simulink model "mrefrobotarm_modified_previous_y_previous_ref"  (R2018b)
settings: Solver=FixedStepAuto  StartTime=0.0  StopTime=60  RelTol=1e-3  AbsTol=1e-6
undefined symbols (not defined in the file or in its folder): sfunxy2
libraries: neural x301, simulink x1
(part 9 of 10)

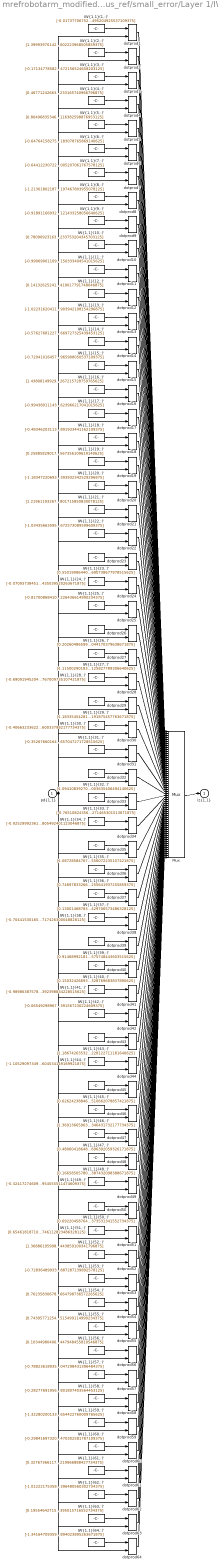
== system mrefrobotarm_modified_previous_y_previous_ref/small_error/Layer 1/IW{1,1} ==
  "pd{1,1}" : Inport  PortDimensions=8
      mask Display: e = 0.06;c1 = [120 230 180]/255;c2 = ([120 230 180]+0)/(256+128);c3 = ([120 230 180]+128)/(256+128);patch([0 1 1 0],[0 0 1 1],c1);patch([0 1 1 1-e 1-e 0+e],[0 0 1 1-e 0+e 0+e],c2);patch([0 0 1 1-e 0+e 0+e],[0 1 1 1-e 1-e 0+e],c3);plot([0 1 1 0 0],[0 0 1 1 0]);
  "IW{1,1}(1,:)'" : Constant  Value=[-0.017377067526509477890517274545345571823418140411376953125;-0.034011354582700097093361790712151560001075267791748046875;0.05439770936445220694821500728721730411052703857421875;-0.0629009283471842761681358524583629332482814788818359375;-2.987224863746458680680007091723382472991943359375;-0.2272943137249578138270322824610047973692417144775390625;0.038579930489393156334276824281914741732180118560791015625;-0.1025768959590427353845143443322740495204925537109375]
      mask Display: e = 0.06;c1 = [120 150 230]/255;c2 = ([120 150 230]+0)/383;c3 = ([120 150 230]+128)/383;patch([0 1 1 0],[0 0 1 1],c1);patch([0 1 1 1-e 1-e 0+e],[0 0 1 1-e 0+e 0+e],c2);patch([0 0 1 1-e 0+e 0+e],[0 1 1 1-e 1-e 0+e],c3);plot([0 1 1 0 0],[0 0 1 1 0]);disp('Weights');
  "IW{1,1}(10,:)'" : Constant  Value=[0.7809092316347172602064574675750918686389923095703125;0.09000232433482556471115998419918469153344631195068359375;-1.0678670373399123949553768397890962660312652587890625;-0.46394015522004983242965181489125825464725494384765625;-0.9896990789374815467027701743063516914844512939453125;-1.3552014415576343342451082207844592630863189697265625;-0.179686656791558874157743730393121950328350067138671875;-0.448255149939543795500895839722943492233753204345703125]
      mask Display: e = 0.06;c1 = [120 150 230]/255;c2 = ([120 150 230]+0)/383;c3 = ([120 150 230]+128)/383;patch([0 1 1 0],[0 0 1 1],c1);patch([0 1 1 1-e 1-e 0+e],[0 0 1 1-e 0+e 0+e],c2);patch([0 0 1 1-e 0+e 0+e],[0 1 1 1-e 1-e 0+e],c3);plot([0 1 1 0 0],[0 0 1 1 0]);disp('Weights');
  "IW{1,1}(11,:)'" : Constant  Value=[-0.99069001109756549272589154497836716473102569580078125;-0.10428566072279556176116699361955397762358188629150390625;0.55618964752205457546807565449853427708148956298828125;0.68297232673513941225706957993679679930210113525390625;-0.248998068763353452848008373621269129216670989990234375;0.644201394846871888688610852113924920558929443359375;1.25138751592991059879977910895831882953643798828125;-1.4140254443841655529467971064150333404541015625]
      mask Display: e = 0.06;c1 = [120 150 230]/255;c2 = ([120 150 230]+0)/383;c3 = ([120 150 230]+128)/383;patch([0 1 1 0],[0 0 1 1],c1);patch([0 1 1 1-e 1-e 0+e],[0 0 1 1-e 0+e 0+e],c2);patch([0 0 1 1-e 0+e 0+e],[0 1 1 1-e 1-e 0+e],c3);plot([0 1 1 0 0],[0 0 1 1 0]);disp('Weights');
  "IW{1,1}(12,:)'" : Constant  Value=[0.1413262524196326752612407062770216725766658782958984375;-0.6047035889340335312880370111088268458843231201171875;0.381641363428228796994545746201765723526477813720703125;0.84755222293533816202426578456652350723743438720703125;0.041896191821087412632262925171744427643716335296630859375;-1.3393596111062613385200847915257327258586883544921875;-1.16826698005478224473563386709429323673248291015625;-0.51017323607084985592763359818491153419017791748046875]
      mask Display: e = 0.06;c1 = [120 150 230]/255;c2 = ([120 150 230]+0)/383;c3 = ([120 150 230]+128)/383;patch([0 1 1 0],[0 0 1 1],c1);patch([0 1 1 1-e 1-e 0+e],[0 0 1 1-e 0+e 0+e],c2);patch([0 0 1 1-e 0+e 0+e],[0 1 1 1-e 1-e 0+e],c3);plot([0 1 1 0 0],[0 0 1 1 0]);disp('Weights');
  "IW{1,1}(13,:)'" : Constant  Value=[-1.0223162041134503663641908133286051452159881591796875;0.360795024277329456907636995310895144939422607421875;0.83528351858334992652288519821013323962688446044921875;-0.419973501162595186375625644359388388693332672119140625;-0.91936716478895308402030650540837086737155914306640625;-0.745110801710211045900678072939626872539520263671875;0.66761104678762228648025711663649417459964752197265625;1.0867368236477321641331172941136173903942108154296875]
      mask Display: e = 0.06;c1 = [120 150 230]/255;c2 = ([120 150 230]+0)/383;c3 = ([120 150 230]+128)/383;patch([0 1 1 0],[0 0 1 1],c1);patch([0 1 1 1-e 1-e 0+e],[0 0 1 1-e 0+e 0+e],c2);patch([0 0 1 1-e 0+e 0+e],[0 1 1 1-e 1-e 0+e],c3);plot([0 1 1 0 0],[0 0 1 1 0]);disp('Weights');
  "IW{1,1}(14,:)'" : Constant  Value=[-0.57627681227857741053099971395567990839481353759765625;0.857909167421744722759058277006261050701141357421875;-0.94860344887297232130407564909546636044979095458984375;-0.951059353750250746628580600372515618801116943359375;-0.08236091843453390015650228406229871325194835662841796875;-1.197742094847008775815311309997923672199249267578125;1.2108252364446354665261651462060399353504180908203125;0.157912941676574991589632190880365669727325439453125]
      mask Display: e = 0.06;c1 = [120 150 230]/255;c2 = ([120 150 230]+0)/383;c3 = ([120 150 230]+128)/383;patch([0 1 1 0],[0 0 1 1],c1);patch([0 1 1 1-e 1-e 0+e],[0 0 1 1-e 0+e 0+e],c2);patch([0 0 1 1-e 0+e 0+e],[0 1 1 1-e 1-e 0+e],c3);plot([0 1 1 0 0],[0 0 1 1 0]);disp('Weights');
  "IW{1,1}(15,:)'" : Constant  Value=[-0.7204101645789158236965477044577710330486297607421875;0.6308160303046788097702801678678952157497406005859375;0.423721818187184962045677139030885882675647735595703125;1.0038491536260936154434375566779635846614837646484375;-0.883054705141663287548681182670406997203826904296875;0.58133530731886706721667223973781801760196685791015625;-1.0898604085723462286949825283954851329326629638671875;0.75502926087022037560103626674390397965908050537109375]
      mask Display: e = 0.06;c1 = [120 150 230]/255;c2 = ([120 150 230]+0)/383;c3 = ([120 150 230]+128)/383;patch([0 1 1 0],[0 0 1 1],c1);patch([0 1 1 1-e 1-e 0+e],[0 0 1 1-e 0+e 0+e],c2);patch([0 0 1 1-e 0+e 0+e],[0 1 1 1-e 1-e 0+e],c3);plot([0 1 1 0 0],[0 0 1 1 0]);disp('Weights');
  "IW{1,1}(16,:)'" : Constant  Value=[1.4380814992902493099080629690433852374553680419921875;-0.76504143837121485471897130992147140204906463623046875;0.091006162532383749752540325062000192701816558837890625;1.083412609067099463544536774861626327037811279296875;-0.63205437136288289412533458744292147457599639892578125;-0.023231907766419000738178368692388175986707210540771484375;-0.38486268286379610170655496403924189507961273193359375;0.97191291146138658607611660045222379267215728759765625]
      mask Display: e = 0.06;c1 = [120 150 230]/255;c2 = ([120 150 230]+0)/383;c3 = ([120 150 230]+128)/383;patch([0 1 1 0],[0 0 1 1],c1);patch([0 1 1 1-e 1-e 0+e],[0 0 1 1-e 0+e 0+e],c2);patch([0 0 1 1-e 0+e 0+e],[0 1 1 1-e 1-e 0+e],c3);plot([0 1 1 0 0],[0 0 1 1 0]);disp('Weights');
  "IW{1,1}(17,:)'" : Constant  Value=[-0.99438911143919117563427789718843996524810791015625;1.1800184823356942853678219762514345347881317138671875;0.96225693879916296413767895501223392784595489501953125;0.92922137731835563467797101111500523984432220458984375;-0.165351050339907879038747751110349781811237335205078125;-0.92189358845869495695524165057577192783355712890625;-0.7329222503569459146177678121603094041347503662109375;-0.386713897740563139482361521004349924623966217041015625]
      mask Display: e = 0.06;c1 = [120 150 230]/255;c2 = ([120 150 230]+0)/383;c3 = ([120 150 230]+128)/383;patch([0 1 1 0],[0 0 1 1],c1);patch([0 1 1 1-e 1-e 0+e],[0 0 1 1-e 0+e 0+e],c2);patch([0 0 1 1-e 0+e 0+e],[0 1 1 1-e 1-e 0+e],c3);plot([0 1 1 0 0],[0 0 1 1 0]);disp('Weights');
  "IW{1,1}(18,:)'" : Constant  Value=[-0.48346203113266172923800922944792546331882476806640625;0.71561240921933866321325012904708273708820343017578125;0.2763669805789514821725560977938584983348846435546875;0.1785391777356719333891277301518130116164684295654296875;-1.282476848547498438080083360546268522739410400390625;-0.345188333939475733291857295625959523022174835205078125;-0.485833446458430129322181301176897250115871429443359375;0.37699947906613962000932360751903615891933441162109375]
      mask Display: e = 0.06;c1 = [120 150 230]/255;c2 = ([120 150 230]+0)/383;c3 = ([120 150 230]+128)/383;patch([0 1 1 0],[0 0 1 1],c1);patch([0 1 1 1-e 1-e 0+e],[0 0 1 1-e 0+e 0+e],c2);patch([0 0 1 1-e 0+e 0+e],[0 1 1 1-e 1-e 0+e],c3);plot([0 1 1 0 0],[0 0 1 1 0]);disp('Weights');
  "IW{1,1}(19,:)'" : Constant  Value=[0.25885829017035144605785035309963859617710113525390625;-0.75860387169028531406667070768889971077442169189453125;1.168586248003583794030646458850242197513580322265625;0.108415735019206482814269065784174017608165740966796875;-1.0403518157121827147904014054802246391773223876953125;0.227217134884770410874210710971965454518795013427734375;-0.1707771036802909758733903800020925700664520263671875;-1.05888387189785504460814991034567356109619140625]
      mask Display: e = 0.06;c1 = [120 150 230]/255;c2 = ([120 150 230]+0)/383;c3 = ([120 150 230]+128)/383;patch([0 1 1 0],[0 0 1 1],c1);patch([0 1 1 1-e 1-e 0+e],[0 0 1 1-e 0+e 0+e],c2);patch([0 0 1 1-e 0+e 0+e],[0 1 1 1-e 1-e 0+e],c3);plot([0 1 1 0 0],[0 0 1 1 0]);disp('Weights');
  "IW{1,1}(2,:)'" : Constant  Value=[1.399939701424660842832281559822149574756622314453125;1.1970420723626855608046071210992522537708282470703125;-1.2136352199150628461410406089271418750286102294921875;-0.52562314227074813377527107149944640696048736572265625;-0.04503930323055231610407389553074608556926250457763671875;0.83699176817769738168095727814943529665470123291015625;0.2363093463990357523396568240059423260390758514404296875;-0.244408544667858718124620054368278943002223968505859375]
      mask Display: e = 0.06;c1 = [120 150 230]/255;c2 = ([120 150 230]+0)/383;c3 = ([120 150 230]+128)/383;patch([0 1 1 0],[0 0 1 1],c1);patch([0 1 1 1-e 1-e 0+e],[0 0 1 1-e 0+e 0+e],c2);patch([0 0 1 1-e 0+e 0+e],[0 1 1 1-e 1-e 0+e],c3);plot([0 1 1 0 0],[0 0 1 1 0]);disp('Weights');
  "IW{1,1}(20,:)'" : Constant  Value=[-1.18347220693401045110704217222519218921661376953125;0.766009156958994186226163947139866650104522705078125;-1.0467062449262838352836979538551531732082366943359375;0.6851787478277435727846977897570468485355377197265625;-0.58848967369292604079333841582410968840122222900390625;0.8268949957131475070326587228919379413127899169921875;-0.8104681829608697540834327810443937778472900390625;0.20686385705200993623265048881876282393932342529296875]
      mask Display: e = 0.06;c1 = [120 150 230]/255;c2 = ([120 150 230]+0)/383;c3 = ([120 150 230]+128)/383;patch([0 1 1 0],[0 0 1 1],c1);patch([0 1 1 1-e 1-e 0+e],[0 0 1 1-e 0+e 0+e],c2);patch([0 0 1 1-e 0+e 0+e],[0 1 1 1-e 1-e 0+e],c3);plot([0 1 1 0 0],[0 0 1 1 0]);disp('Weights');
  "IW{1,1}(21,:)'" : Constant  Value=[1.219611932677147958514751735492609441280364990234375;-0.2179986107852489862768408102056127972900867462158203125;0.6892814533111317754077163044712506234645843505859375;1.2392353114451151174790766162914223968982696533203125;-0.59287581991320070784468043711967766284942626953125;-0.1463361983944102828747446665147435851395130157470703125;0.443878498993484249535157459831680171191692352294921875;-1.227012857090613806576584465801715850830078125]
      mask Display: e = 0.06;c1 = [120 150 230]/255;c2 = ([120 150 230]+0)/383;c3 = ([120 150 230]+128)/383;patch([0 1 1 0],[0 0 1 1],c1);patch([0 1 1 1-e 1-e 0+e],[0 0 1 1-e 0+e 0+e],c2);patch([0 0 1 1-e 0+e 0+e],[0 1 1 1-e 1-e 0+e],c3);plot([0 1 1 0 0],[0 0 1 1 0]);disp('Weights');
  "IW{1,1}(22,:)'" : Constant  Value=[-1.034356635952660585786588853807188570499420166015625;-0.2124491322472994159209491726869600825011730194091796875;0.90244981411305413843138012452982366085052490234375;-0.049504035624847932128833605247564264573156833648681640625;-0.72694661999179366329570939342374913394451141357421875;1.1420952393322547635534647270105779170989990234375;1.1682637955611234747976823200588114559650421142578125;-0.0639384741576127790807504425174556672573089599609375]
      mask Display: e = 0.06;c1 = [120 150 230]/255;c2 = ([120 150 230]+0)/383;c3 = ([120 150 230]+128)/383;patch([0 1 1 0],[0 0 1 1],c1);patch([0 1 1 1-e 1-e 0+e],[0 0 1 1-e 0+e 0+e],c2);patch([0 0 1 1-e 0+e 0+e],[0 1 1 1-e 1-e 0+e],c3);plot([0 1 1 0 0],[0 0 1 1 0]);disp('Weights');
  "IW{1,1}(23,:)'" : Constant  Value=[0.55019086440172249030666762337205000221729278564453125;-1.0819049497302071216608965187333524227142333984375;0.9266808173211398269586425158195197582244873046875;-1.187292059671042121493655940867029130458831787109375;0.344402574037255326810935684989090077579021453857421875;0.956062103710445310156273990287445485591888427734375;0.847530837657149316299864949542097747325897216796875;-0.406884376651751422659941681558848358690738677978515625]
      mask Display: e = 0.06;c1 = [120 150 230]/255;c2 = ([120 150 230]+0)/383;c3 = ([120 150 230]+128)/383;patch([0 1 1 0],[0 0 1 1],c1);patch([0 1 1 1-e 1-e 0+e],[0 0 1 1-e 0+e 0+e],c2);patch([0 0 1 1-e 0+e 0+e],[0 1 1 1-e 1-e 0+e],c3);plot([0 1 1 0 0],[0 0 1 1 0]);disp('Weights');
  "IW{1,1}(24,:)'" : Constant  Value=[-0.0709373845187223073249782601124024949967861175537109375;-1.121192740111934593727482933900319039821624755859375;0.30768431517374061900937931568478234112262725830078125;-1.445687820244011323467248075758107006549835205078125;-0.69216758774098929851703587701194919645786285400390625;1.24765852733028026477768435142934322357177734375;-0.027293636765880140149231891655290382914245128631591796875;0.08892851627873710196325873766909353435039520263671875]
      mask Display: e = 0.06;c1 = [120 150 230]/255;c2 = ([120 150 230]+0)/383;c3 = ([120 150 230]+128)/383;patch([0 1 1 0],[0 0 1 1],c1);patch([0 1 1 1-e 1-e 0+e],[0 0 1 1-e 0+e 0+e],c2);patch([0 0 1 1-e 0+e 0+e],[0 1 1 1-e 1-e 0+e],c3);plot([0 1 1 0 0],[0 0 1 1 0]);disp('Weights');
  "IW{1,1}(25,:)'" : Constant  Value=[-0.817008684104527649338933770195581018924713134765625;0.09009373381231032540394920715698390267789363861083984375;-0.728342621944587431670470323297195136547088623046875;-0.9599684782971167340548390711774118244647979736328125;1.115180526327934185104595599113963544368743896484375;1.0179637090492612561121177350287325680255889892578125;0.59465668759401413279164216874050907790660858154296875;0.64504891126972674353368120137020014226436614990234375]
      mask Display: e = 0.06;c1 = [120 150 230]/255;c2 = ([120 150 230]+0)/383;c3 = ([120 150 230]+128)/383;patch([0 1 1 0],[0 0 1 1],c1);patch([0 1 1 1-e 1-e 0+e],[0 0 1 1-e 0+e 0+e],c2);patch([0 0 1 1-e 0+e 0+e],[0 1 1 1-e 1-e 0+e],c3);plot([0 1 1 0 0],[0 0 1 1 0]);disp('Weights');
  "IW{1,1}(26,:)'" : Constant  Value=[0.2026048659954693687001991975193959660828113555908203125;-0.89940805135049206597841475741006433963775634765625;-0.588853479835137694209379333187825977802276611328125;0.30103005113216896315719850463210605084896087646484375;0.367424398316437195166628271181252785027027130126953125;-1.28156467127469841926767912809737026691436767578125;1.176220308682861315219270181842148303985595703125;-0.93983343655070228361836370822857134044170379638671875]
      mask Display: e = 0.06;c1 = [120 150 230]/255;c2 = ([120 150 230]+0)/383;c3 = ([120 150 230]+128)/383;patch([0 1 1 0],[0 0 1 1],c1);patch([0 1 1 1-e 1-e 0+e],[0 0 1 1-e 0+e 0+e],c2);patch([0 0 1 1-e 0+e 0+e],[0 1 1 1-e 1-e 0+e],c3);plot([0 1 1 0 0],[0 0 1 1 0]);disp('Weights');
  "IW{1,1}(27,:)'" : Constant  Value=[1.1150029018346951925622079215827398002147674560546875;-0.107338087221813094362943274973076768219470977783203125;1.183594109106976599576910302857868373394012451171875;-1.039098304448061949045722940354607999324798583984375;0.74480545136070486211821162214619107544422149658203125;0.61027453990553237606064840292674489319324493408203125;0.32286624411939979228947095180046744644641876220703125;0.723064851875764080801900490769185125827789306640625]
      mask Display: e = 0.06;c1 = [120 150 230]/255;c2 = ([120 150 230]+0)/383;c3 = ([120 150 230]+128)/383;patch([0 1 1 0],[0 0 1 1],c1);patch([0 1 1 1-e 1-e 0+e],[0 0 1 1-e 0+e 0+e],c2);patch([0 0 1 1-e 0+e 0+e],[0 1 1 1-e 1-e 0+e],c3);plot([0 1 1 0 0],[0 0 1 1 0]);disp('Weights');
  "IW{1,1}(28,:)'" : Constant  Value=[-0.690919452047221938073562341742217540740966796875;-0.55427096371533968177658380227512679994106292724609375;0.82704898973293572428389097694889642298221588134765625;0.6540987147296088988213114134850911796092987060546875;1.2194524981285737030844984474242664873600006103515625;-1.213898767528181821262478479184210300445556640625;0.1279128539486860116625166483572684228420257568359375;-0.3054058139714264097364093686337582767009735107421875]
      mask Display: e = 0.06;c1 = [120 150 230]/255;c2 = ([120 150 230]+0)/383;c3 = ([120 150 230]+128)/383;patch([0 1 1 0],[0 0 1 1],c1);patch([0 1 1 1-e 1-e 0+e],[0 0 1 1-e 0+e 0+e],c2);patch([0 0 1 1-e 0+e 0+e],[0 1 1 1-e 1-e 0+e],c3);plot([0 1 1 0 0],[0 0 1 1 0]);disp('Weights');
  "IW{1,1}(29,:)'" : Constant  Value=[1.1833545428174867542026049704873003065586090087890625;-0.37617049447265127337658441319945268332958221435546875;0.08312849877137044873887106177789974026381969451904296875;-0.65728646232727550025032314806594513356685638427734375;-1.1565053035930912272988280165009200572967529296875;-1.2174699300370388499459295417182147502899169921875;-0.58854994883035083308442381166969425976276397705078125;-0.588524694941269910231085304985754191875457763671875]
      mask Display: e = 0.06;c1 = [120 150 230]/255;c2 = ([120 150 230]+0)/383;c3 = ([120 150 230]+128)/383;patch([0 1 1 0],[0 0 1 1],c1);patch([0 1 1 1-e 1-e 0+e],[0 0 1 1-e 0+e 0+e],c2);patch([0 0 1 1-e 0+e 0+e],[0 1 1 1-e 1-e 0+e],c3);plot([0 1 1 0 0],[0 0 1 1 0]);disp('Weights');
  "IW{1,1}(3,:)'" : Constant  Value=[-0.1713477858219417948593132905443781055510044097900390625;-1.0375213286223470277036540210247039794921875;-1.1152868460490157342945849450188688933849334716796875;-0.56009756828457113453367810507188551127910614013671875;-0.467727208222955825878131008721538819372653961181640625;0.067216770819887028398653683325392194092273712158203125;0.1100353684041793511649842685073963366448879241943359375;1.2683448907835963570533976962906308472156524658203125]
      mask Display: e = 0.06;c1 = [120 150 230]/255;c2 = ([120 150 230]+0)/383;c3 = ([120 150 230]+128)/383;patch([0 1 1 0],[0 0 1 1],c1);patch([0 1 1 1-e 1-e 0+e],[0 0 1 1-e 0+e 0+e],c2);patch([0 0 1 1-e 0+e 0+e],[0 1 1 1-e 1-e 0+e],c3);plot([0 1 1 0 0],[0 0 1 1 0]);disp('Weights');
  "IW{1,1}(30,:)'" : Constant  Value=[-0.406632336224892421139287534970208071172237396240234375;-0.071691479079252662387489181128330528736114501953125;0.953885436919628570962004232569597661495208740234375;-0.370319891288378999494312893148162402212619781494140625;-0.350997147144751997505096596796647645533084869384765625;-0.76124062166233696924422247320762835443019866943359375;0.1624752428543290161400136639713309705257415771484375;-0.67908939070850971031489962115301750600337982177734375]
      mask Display: e = 0.06;c1 = [120 150 230]/255;c2 = ([120 150 230]+0)/383;c3 = ([120 150 230]+128)/383;patch([0 1 1 0],[0 0 1 1],c1);patch([0 1 1 1-e 1-e 0+e],[0 0 1 1-e 0+e 0+e],c2);patch([0 0 1 1-e 0+e 0+e],[0 1 1 1-e 1-e 0+e],c3);plot([0 1 1 0 0],[0 0 1 1 0]);disp('Weights');
  "IW{1,1}(31,:)'" : Constant  Value=[-0.352676601643936715735350162503891624510288238525390625;-0.67670082960554001072495111657190136611461639404296875;0.41025695896948521923519592746743001043796539306640625;1.158666227866344211605564851197414100170135498046875;-0.75282230283853579511088582876254804432392120361328125;0.5066310090314090075480635277926921844482421875;1.0078083027607360744326570056728087365627288818359375;1.2799313545316393092576845447183586657047271728515625]
      mask Display: e = 0.06;c1 = [120 150 230]/255;c2 = ([120 150 230]+0)/383;c3 = ([120 150 230]+128)/383;patch([0 1 1 0],[0 0 1 1],c1);patch([0 1 1 1-e 1-e 0+e],[0 0 1 1-e 0+e 0+e],c2);patch([0 0 1 1-e 0+e 0+e],[0 1 1 1-e 1-e 0+e],c3);plot([0 1 1 0 0],[0 0 1 1 0]);disp('Weights');
  "IW{1,1}(32,:)'" : Constant  Value=[1.09410839270226034614097443409264087677001953125;0.128116507297960591227337090458604507148265838623046875;1.1755906192236746932167079648934304714202880859375;0.6401292036956942599346120914560742676258087158203125;-0.93505576990294059225306000371347181499004364013671875;-0.1029298762998116512079604945029132068157196044921875;1.000494005965565147420193170546554028987884521484375;-0.82294403689114192790299284752109088003635406494140625]
      mask Display: e = 0.06;c1 = [120 150 230]/255;c2 = ([120 150 230]+0)/383;c3 = ([120 150 230]+128)/383;patch([0 1 1 0],[0 0 1 1],c1);patch([0 1 1 1-e 1-e 0+e],[0 0 1 1-e 0+e 0+e],c2);patch([0 0 1 1-e 0+e 0+e],[0 1 1 1-e 1-e 0+e],c3);plot([0 1 1 0 0],[0 0 1 1 0]);disp('Weights');
  "IW{1,1}(33,:)'" : Constant  Value=[-0.76510824356968576420712224717135541141033172607421875;0.462713514982440177192302144248969852924346923828125;0.771388322645548907274815064738504588603973388671875;-0.461437899328466960557904030792997218668460845947265625;-0.448411725015751161382837608471163548529148101806640625;-0.83972247550148326755703465096303261816501617431640625;-1.44743644356056311295333216548897325992584228515625;-0.46562703172859698508290193785796873271465301513671875]
      mask Display: e = 0.06;c1 = [120 150 230]/255;c2 = ([120 150 230]+0)/383;c3 = ([120 150 230]+128)/383;patch([0 1 1 0],[0 0 1 1],c1);patch([0 1 1 1-e 1-e 0+e],[0 0 1 1-e 0+e 0+e],c2);patch([0 0 1 1-e 0+e 0+e],[0 1 1 1-e 1-e 0+e],c3);plot([0 1 1 0 0],[0 0 1 1 0]);disp('Weights');
  "IW{1,1}(34,:)'" : Constant  Value=[-0.92529992361391133481873794153216294944286346435546875;-0.5525505265953547517909782982314936816692352294921875;1.451139064894599872701519416295923292636871337890625;-1.2992793939354994048329672295949421823024749755859375;0.2768254207230336216838395557715557515621185302734375;0.3264662260228965440234105699346400797367095947265625;-0.0239728882122877164084773227159530506469309329986572265625;0.440115141255702890799028637047740630805492401123046875]
      mask Display: e = 0.06;c1 = [120 150 230]/255;c2 = ([120 150 230]+0)/383;c3 = ([120 150 230]+128)/383;patch([0 1 1 0],[0 0 1 1],c1);patch([0 1 1 1-e 1-e 0+e],[0 0 1 1-e 0+e 0+e],c2);patch([0 0 1 1-e 0+e 0+e],[0 1 1 1-e 1-e 0+e],c3);plot([0 1 1 0 0],[0 0 1 1 0]);disp('Weights');
  "IW{1,1}(35,:)'" : Constant  Value=[1.08728584767184965897968140779994428157806396484375;-0.57920862423610219860137249270337633788585662841796875;0.31020421933113606627330227638594806194305419921875;0.22658140199870924202940614122780971229076385498046875;1.1898272093793667014693937744596041738986968994140625;-0.297311158932645813735007322975434362888336181640625;1.0269246501725657338965902454219758510589599609375;-0.776882115177407239769991065259091556072235107421875]
      mask Display: e = 0.06;c1 = [120 150 230]/255;c2 = ([120 150 230]+0)/383;c3 = ([120 150 230]+128)/383;patch([0 1 1 0],[0 0 1 1],c1);patch([0 1 1 1-e 1-e 0+e],[0 0 1 1-e 0+e 0+e],c2);patch([0 0 1 1-e 0+e 0+e],[0 1 1 1-e 1-e 0+e],c3);plot([0 1 1 0 0],[0 0 1 1 0]);disp('Weights');
  "IW{1,1}(36,:)'" : Constant  Value=[0.7469783326675238921410482362261973321437835693359375;-0.5590277268773051755346159552573226392269134521484375;-0.286969937577315870047556245481246151030063629150390625;-0.90586134408508822701833196333609521389007568359375;1.0883679300743620554925428223214112222194671630859375;0.62737343497663611291415008963667787611484527587890625;0.85802125276730600855756847522570751607418060302734375;-0.684565734927884417260202098987065255641937255859375]
      mask Display: e = 0.06;c1 = [120 150 230]/255;c2 = ([120 150 230]+0)/383;c3 = ([120 150 230]+128)/383;patch([0 1 1 0],[0 0 1 1],c1);patch([0 1 1 1-e 1-e 0+e],[0 0 1 1-e 0+e 0+e],c2);patch([0 0 1 1-e 0+e 0+e],[0 1 1 1-e 1-e 0+e],c3);plot([0 1 1 0 0],[0 0 1 1 0]);disp('Weights');
  "IW{1,1}(37,:)'" : Constant  Value=[0.13001468783774250415063988839392550289630889892578125;-0.10423695612336414395571182467392645776271820068359375;-0.75606516155219993802205635802238248288631439208984375;0.316519047291030364288388909699278883635997772216796875;1.34193595484161232178621503408066928386688232421875;-1.084924692783397315309912301017902791500091552734375;1.112713738288932940889708333997987210750579833984375;-0.73699046018989122774911493252147920429706573486328125]
      mask Display: e = 0.06;c1 = [120 150 230]/255;c2 = ([120 150 230]+0)/383;c3 = ([120 150 230]+128)/383;patch([0 1 1 0],[0 0 1 1],c1);patch([0 1 1 1-e 1-e 0+e],[0 0 1 1-e 0+e 0+e],c2);patch([0 0 1 1-e 0+e 0+e],[0 1 1 1-e 1-e 0+e],c3);plot([0 1 1 0 0],[0 0 1 1 0]);disp('Weights');
  "IW{1,1}(38,:)'" : Constant  Value=[-0.70441530165524268713994615609408356249332427978515625;-1.1872343925763682026541800951235927641391754150390625;0.4135662628199490153946271675522439181804656982421875;0.8929315806927340393173153643147088587284088134765625;-1.0687381637064550243820804098504595458507537841796875;-0.35949622186414875724125295164412818849086761474609375;0.98752354627134308895364256386528722941875457763671875;-0.08749210146199799809085817514642258174717426300048828125]
      mask Display: e = 0.06;c1 = [120 150 230]/255;c2 = ([120 150 230]+0)/383;c3 = ([120 150 230]+128)/383;patch([0 1 1 0],[0 0 1 1],c1);patch([0 1 1 1-e 1-e 0+e],[0 0 1 1-e 0+e 0+e],c2);patch([0 0 1 1-e 0+e 0+e],[0 1 1 1-e 1-e 0+e],c3);plot([0 1 1 0 0],[0 0 1 1 0]);disp('Weights');
  "IW{1,1}(39,:)'" : Constant  Value=[0.9146899218170114753689858844154514372348785400390625;-0.9226021049054173861492245123372413218021392822265625;1.1143145008042842913908998525585047900676727294921875;-0.2493759667926167267193449106343905441462993621826171875;0.4824314841955172905585413900553248822689056396484375;1.3434150904225876654862759096431545913219451904296875;0.385282691103394636655821159365586936473846435546875;0.405601930914338437705879414352239109575748443603515625]
      mask Display: e = 0.06;c1 = [120 150 230]/255;c2 = ([120 150 230]+0)/383;c3 = ([120 150 230]+128)/383;patch([0 1 1 0],[0 0 1 1],c1);patch([0 1 1 1-e 1-e 0+e],[0 0 1 1-e 0+e 0+e],c2);patch([0 0 1 1-e 0+e 0+e],[0 1 1 1-e 1-e 0+e],c3);plot([0 1 1 0 0],[0 0 1 1 0]);disp('Weights');
  "IW{1,1}(4,:)'" : Constant  Value=[0.4677124266352006287661424721591174602508544921875;1.179319538639485909214954517665319144725799560546875;0.1190787283441280541840257001240388490259647369384765625;-0.6254155655293782700709925848059356212615966796875;1.2288866023152780204696910004713572561740875244140625;-0.416970767892102467389037201428436674177646636962890625;-1.15040107186096118851992287090979516506195068359375;-0.81776347676258598351495265887933783233165740966796875]
      mask Display: e = 0.06;c1 = [120 150 230]/255;c2 = ([120 150 230]+0)/383;c3 = ([120 150 230]+128)/383;patch([0 1 1 0],[0 0 1 1],c1);patch([0 1 1 1-e 1-e 0+e],[0 0 1 1-e 0+e 0+e],c2);patch([0 0 1 1-e 0+e 0+e],[0 1 1 1-e 1-e 0+e],c3);plot([0 1 1 0 0],[0 0 1 1 0]);disp('Weights');
  "IW{1,1}(40,:)'" : Constant  Value=[0.150324266934207917412180677274591289460659027099609375;0.92184916947260731046043247260968200862407684326171875;-0.5770663616818143548670150266843847930431365966796875;0.68991099346128936797839514838415198028087615966796875;0.97393249350662258745359167733113281428813934326171875;-1.1663080517874846453452164496411569416522979736328125;-0.6430241425634088958673828528844751417636871337890625;-0.256736913654239951032565159039222635328769683837890625]
      mask Display: e = 0.06;c1 = [120 150 230]/255;c2 = ([120 150 230]+0)/383;c3 = ([120 150 230]+128)/383;patch([0 1 1 0],[0 0 1 1],c1);patch([0 1 1 1-e 1-e 0+e],[0 0 1 1-e 0+e 0+e],c2);patch([0 0 1 1-e 0+e 0+e],[0 1 1 1-e 1-e 0+e],c3);plot([0 1 1 0 0],[0 0 1 1 0]);disp('Weights');
  "IW{1,1}(41,:)'" : Constant  Value=[-0.989863875785313762634132217499427497386932373046875;0.78649592905462906156088820353033952414989471435546875;0.92692012405395940444208235931000672280788421630859375;-0.69214885574553275393583362529170699417591094970703125;-1.0158275700337997538014178644516505300998687744140625;-0.1565018125136950211118147535671596415340900421142578125;-0.488561324717758704849757123156450688838958740234375;-0.6245164074136353438149171779514290392398834228515625]
      mask Display: e = 0.06;c1 = [120 150 230]/255;c2 = ([120 150 230]+0)/383;c3 = ([120 150 230]+128)/383;patch([0 1 1 0],[0 0 1 1],c1);patch([0 1 1 1-e 1-e 0+e],[0 0 1 1-e 0+e 0+e],c2);patch([0 0 1 1-e 0+e 0+e],[0 1 1 1-e 1-e 0+e],c3);plot([0 1 1 0 0],[0 0 1 1 0]);disp('Weights');
  "IW{1,1}(42,:)'" : Constant  Value=[-0.0654929896709634251639187141336151398718357086181640625;-0.126590018741224052956084733523312024772167205810546875;0.676568223684226754954806892783381044864654541015625;0.1119224689992519561343442546785809099674224853515625;0.77417817970255342618912663965602405369281768798828125;0.1666440179828475864898251757040270604193210601806640625;-0.66100299728717593072957470212713815271854400634765625;-0.05042216511042417470545018431948847137391567230224609375]
      mask Display: e = 0.06;c1 = [120 150 230]/255;c2 = ([120 150 230]+0)/383;c3 = ([120 150 230]+128)/383;patch([0 1 1 0],[0 0 1 1],c1);patch([0 1 1 1-e 1-e 0+e],[0 0 1 1-e 0+e 0+e],c2);patch([0 0 1 1-e 0+e 0+e],[0 1 1 1-e 1-e 0+e],c3);plot([0 1 1 0 0],[0 0 1 1 0]);disp('Weights');
  "IW{1,1}(43,:)'" : Constant  Value=[1.186742635320275240928822313435375690460205078125;0.72700473977794810576114059585961513221263885498046875;0.2005686019077405901622768169545452110469341278076171875;-0.81089106499427565655224725560401566326618194580078125;-1.1814745165865427889428929120185784995555877685546875;-0.59164267859916386260721310463850386440753936767578125;-0.9012555659763676896290007789502851665019989013671875;-0.37750023621114225935713193393894471228122711181640625]
      mask Display: e = 0.06;c1 = [120 150 230]/255;c2 = ([120 150 230]+0)/383;c3 = ([120 150 230]+128)/383;patch([0 1 1 0],[0 0 1 1],c1);patch([0 1 1 1-e 1-e 0+e],[0 0 1 1-e 0+e 0+e],c2);patch([0 0 1 1-e 0+e 0+e],[0 1 1 1-e 1-e 0+e],c3);plot([0 1 1 0 0],[0 0 1 1 0]);disp('Weights');
  "IW{1,1}(44,:)'" : Constant  Value=[-1.105290973495005601989760180003941059112548828125;-0.32597663112844499355702510001719929277896881103515625;-0.6594988375978301231583600383601151406764984130859375;-0.319229986332627502232384131275466643273830413818359375;1.3534773499650594175136575358919799327850341796875;0.57122266331391546856366403517313301563262939453125;0.8013418587414318228212550820899195969104766845703125;-0.1307407917426086363388293420939589850604534149169921875]
      mask Display: e = 0.06;c1 = [120 150 230]/255;c2 = ([120 150 230]+0)/383;c3 = ([120 150 230]+128)/383;patch([0 1 1 0],[0 0 1 1],c1);patch([0 1 1 1-e 1-e 0+e],[0 0 1 1-e 0+e 0+e],c2);patch([0 0 1 1-e 0+e 0+e],[0 1 1 1-e 1-e 0+e],c3);plot([0 1 1 0 0],[0 0 1 1 0]);disp('Weights');
  "IW{1,1}(45,:)'" : Constant  Value=[0.62624238846817326109572832137928344309329986572265625;0.14703808415278685206573072719038464128971099853515625;0.457398557723452114931461665037204511463642120361328125;0.72188630672245945874010430998168885707855224609375;-0.33557716928372960385473788846866227686405181884765625;0.57064174918386478818632667753263376653194427490234375;-1.4672029223197620151353248729719780385494232177734375;-1.2234915425500012542414651761646382510662078857421875]
      mask Display: e = 0.06;c1 = [120 150 230]/255;c2 = ([120 150 230]+0)/383;c3 = ([120 150 230]+128)/383;patch([0 1 1 0],[0 0 1 1],c1);patch([0 1 1 1-e 1-e 0+e],[0 0 1 1-e 0+e 0+e],c2);patch([0 0 1 1-e 0+e 0+e],[0 1 1 1-e 1-e 0+e],c3);plot([0 1 1 0 0],[0 0 1 1 0]);disp('Weights');
  "IW{1,1}(46,:)'" : Constant  Value=[1.3691366596317637860380500569590367376804351806640625;0.3329397731164618345900407803128473460674285888671875;0.57139335167013782790235154607216827571392059326171875;0.51010398909026000158206670676008798182010650634765625;-1.1097921255095155590453259719652123749256134033203125;-0.73643732777806214517823946152930147945880889892578125;-0.2840819022141121141800113036879338324069976806640625;-1.0006883785963560651310899629606865346431732177734375]
      mask Display: e = 0.06;c1 = [120 150 230]/255;c2 = ([120 150 230]+0)/383;c3 = ([120 150 230]+128)/383;patch([0 1 1 0],[0 0 1 1],c1);patch([0 1 1 1-e 1-e 0+e],[0 0 1 1-e 0+e 0+e],c2);patch([0 0 1 1-e 0+e 0+e],[0 1 1 1-e 1-e 0+e],c3);plot([0 1 1 0 0],[0 0 1 1 0]);disp('Weights');
  "IW{1,1}(47,:)'" : Constant  Value=[0.480604186486641438147415783532778732478618621826171875;0.84422588131719111803619171041646040976047515869140625;0.82453351319982404188380087362020276486873626708984375;-1.18107295599703032706884187064133584499359130859375;1.019371481649084199005983464303426444530487060546875;-0.96232788375230182698061298651737160980701446533203125;-0.6610640726387975174560551749891601502895355224609375;0.339991176458866117826573827187530696392059326171875]
      mask Display: e = 0.06;c1 = [120 150 230]/255;c2 = ([120 150 230]+0)/383;c3 = ([120 150 230]+128)/383;patch([0 1 1 0],[0 0 1 1],c1);patch([0 1 1 1-e 1-e 0+e],[0 0 1 1-e 0+e 0+e],c2);patch([0 0 1 1-e 0+e 0+e],[0 1 1 1-e 1-e 0+e],c3);plot([0 1 1 0 0],[0 0 1 1 0]);disp('Weights');
  "IW{1,1}(48,:)'" : Constant  Value=[0.16658505780300547627348350943066179752349853515625;-0.07588862743271031219283173641088069416582584381103515625;-0.11745889146021588900214993600457091815769672393798828125;0.10806056174435356431740018479104037396609783172607421875;3.46068702604472644424049576628021895885467529296875;0.04341703733599792947028817025056923739612102508544921875;0.435289324953846146204483602559776045382022857666015625;-0.23325230586292178269758323949645273387432098388671875]
      mask Display: e = 0.06;c1 = [120 150 230]/255;c2 = ([120 150 230]+0)/383;c3 = ([120 150 230]+128)/383;patch([0 1 1 0],[0 0 1 1],c1);patch([0 1 1 1-e 1-e 0+e],[0 0 1 1-e 0+e 0+e],c2);patch([0 0 1 1-e 0+e 0+e],[0 1 1 1-e 1-e 0+e],c3);plot([0 1 1 0 0],[0 0 1 1 0]);disp('Weights');
  "IW{1,1}(49,:)'" : Constant  Value=[-0.324172746097600938952609794796444475650787353515625;-1.040872905725482855388008829322643578052520751953125;-1.627380137454742747848968065227381885051727294921875;-0.358118770152060672540272889818879775702953338623046875;0.425375034709552679590416346400161273777484893798828125;-0.630583468276700198629214355605654418468475341796875;0.87327934704026299872481331476592458784580230712890625;0.3660859794185602478222563149756751954555511474609375]
      mask Display: e = 0.06;c1 = [120 150 230]/255;c2 = ([120 150 230]+0)/383;c3 = ([120 150 230]+128)/383;patch([0 1 1 0],[0 0 1 1],c1);patch([0 1 1 1-e 1-e 0+e],[0 0 1 1-e 0+e 0+e],c2);patch([0 0 1 1-e 0+e 0+e],[0 1 1 1-e 1-e 0+e],c3);plot([0 1 1 0 0],[0 0 1 1 0]);disp('Weights');
  "IW{1,1}(5,:)'" : Constant  Value=[0.80496835346537254363141755675314925611019134521484375;0.09846330826343203945771875851278309710323810577392578125;-1.38376904242930010013878927566111087799072265625;-0.2188869464847831569631608772397157736122608184814453125;-0.7628228978433480023113588686101138591766357421875;-0.459195914314611541851007814329932443797588348388671875;0.55615377789827868948435707352473400533199310302734375;0.76675629522494948009381232623127289116382598876953125]
      mask Display: e = 0.06;c1 = [120 150 230]/255;c2 = ([120 150 230]+0)/383;c3 = ([120 150 230]+128)/383;patch([0 1 1 0],[0 0 1 1],c1);patch([0 1 1 1-e 1-e 0+e],[0 0 1 1-e 0+e 0+e],c2);patch([0 0 1 1-e 0+e 0+e],[0 1 1 1-e 1-e 0+e],c3);plot([0 1 1 0 0],[0 0 1 1 0]);disp('Weights');
  "IW{1,1}(50,:)'" : Constant  Value=[0.69220458764794645656337479522335343062877655029296875;-1.193685042063108436849461213569156825542449951171875;0.917288662957973510714282383560203015804290771484375;-0.34810562554271717861098522917018271982669830322265625;1.1522442270627764049351071662385948002338409423828125;-0.74321846129039548234374024104909040033817291259765625;-0.8333227884286376063727175278472714126110076904296875;-0.50881779653028524901259288526489399373531341552734375]
      mask Display: e = 0.06;c1 = [120 150 230]/255;c2 = ([120 150 230]+0)/383;c3 = ([120 150 230]+128)/383;patch([0 1 1 0],[0 0 1 1],c1);patch([0 1 1 1-e 1-e 0+e],[0 0 1 1-e 0+e 0+e],c2);patch([0 0 1 1-e 0+e 0+e],[0 1 1 1-e 1-e 0+e],c3);plot([0 1 1 0 0],[0 0 1 1 0]);disp('Weights');
  "IW{1,1}(51,:)'" : Constant  Value=[0.654618187101493109736338738002814352512359619140625;0.57725558454009651132565750231151469051837921142578125;-0.377185469959709251952517661266028881072998046875;-1.013291811267324593615057892748154699802398681640625;-0.70224794420951008877551657860749401152133941650390625;0.94163301176554659033257621558732353150844573974609375;-0.87173448369511785660534997077775187790393829345703125;1.0589877439578743167913899014820344746112823486328125]
      mask Display: e = 0.06;c1 = [120 150 230]/255;c2 = ([120 150 230]+0)/383;c3 = ([120 150 230]+128)/383;patch([0 1 1 0],[0 0 1 1],c1);patch([0 1 1 1-e 1-e 0+e],[0 0 1 1-e 0+e 0+e],c2);patch([0 0 1 1-e 0+e 0+e],[0 1 1 1-e 1-e 0+e],c3);plot([0 1 1 0 0],[0 0 1 1 0]);disp('Weights');
  "IW{1,1}(52,:)'" : Constant  Value=[1.3688619599808398152873678554897196590900421142578125;-0.50237260656056559326998467440716922283172607421875;1.0203014056071963988614470508764497935771942138671875;1.4401690630730874520537554417387582361698150634765625;-0.134334404109476890365471035693190060555934906005859375;0.63086523561595930775780516341910697519779205322265625;0.10910016859874029082622115538470097817480564117431640625;-0.5603657024301174072178355345386080443859100341796875]
      mask Display: e = 0.06;c1 = [120 150 230]/255;c2 = ([120 150 230]+0)/383;c3 = ([120 150 230]+128)/383;patch([0 1 1 0],[0 0 1 1],c1);patch([0 1 1 1-e 1-e 0+e],[0 0 1 1-e 0+e 0+e],c2);patch([0 0 1 1-e 0+e 0+e],[0 1 1 1-e 1-e 0+e],c3);plot([0 1 1 0 0],[0 0 1 1 0]);disp('Weights');
  "IW{1,1}(53,:)'" : Constant  Value=[-0.7283648993366502732982326051569543778896331787109375;-0.296522662182558682797406390818650834262371063232421875;1.30678063995774973449215394794009625911712646484375;-0.340747658274968057146026012560469098389148712158203125;-0.87947548057460001036389485307154245674610137939453125;0.36407241329327388879022464607260189950466156005859375;-1.40416053120731731951309484429657459259033203125;0.548976410428668515351091627962887287139892578125]
      mask Display: e = 0.06;c1 = [120 150 230]/255;c2 = ([120 150 230]+0)/383;c3 = ([120 150 230]+128)/383;patch([0 1 1 0],[0 0 1 1],c1);patch([0 1 1 1-e 1-e 0+e],[0 0 1 1-e 0+e 0+e],c2);patch([0 0 1 1-e 0+e 0+e],[0 1 1 1-e 1-e 0+e],c3);plot([0 1 1 0 0],[0 0 1 1 0]);disp('Weights');
  "IW{1,1}(54,:)'" : Constant  Value=[0.76235830678807336990843168678111396729946136474609375;-0.263400737160603359843236148662981577217578887939453125;-0.52733492353464661572814975443179719150066375732421875;0.264341887289500920843465792131610214710235595703125;-1.313367287391855153799724575947038829326629638671875;0.364040256891997149324424754013307392597198486328125;0.51766650449105700015905995314824394881725311279296875;1.5137623857976569841099490076885558664798736572265625]
      mask Display: e = 0.06;c1 = [120 150 230]/255;c2 = ([120 150 230]+0)/383;c3 = ([120 150 230]+128)/383;patch([0 1 1 0],[0 0 1 1],c1);patch([0 1 1 1-e 1-e 0+e],[0 0 1 1-e 0+e 0+e],c2);patch([0 0 1 1-e 0+e 0+e],[0 1 1 1-e 1-e 0+e],c3);plot([0 1 1 0 0],[0 0 1 1 0]);disp('Weights');
  "IW{1,1}(55,:)'" : Constant  Value=[0.74395771254309572828589125492726452648639678955078125;-0.16337813680087098777704568419721908867359161376953125;-0.64460345699131005314796993843629024922847747802734375;-0.4674568802613652263033827694016508758068084716796875;-1.1916712358503718238722512978711165487766265869140625;-0.58836195577556937852392593413242138922214508056640625;-0.296193419474662100743245218836818821728229522705078125;-1.0983538205506542251299606505199335515499114990234375]
      mask Display: e = 0.06;c1 = [120 150 230]/255;c2 = ([120 150 230]+0)/383;c3 = ([120 150 230]+128)/383;patch([0 1 1 0],[0 0 1 1],c1);patch([0 1 1 1-e 1-e 0+e],[0 0 1 1-e 0+e 0+e],c2);patch([0 0 1 1-e 0+e 0+e],[0 1 1 1-e 1-e 0+e],c3);plot([0 1 1 0 0],[0 0 1 1 0]);disp('Weights');
  "IW{1,1}(56,:)'" : Constant  Value=[0.103449804069278672447040889892377890646457672119140625;-0.11265942328387247572951679330799379386007785797119140625;0.5581356619217212600148059209459461271762847900390625;-0.37085152996991876950261257661622948944568634033203125;1.74270939706490590737075763172470033168792724609375;0.22202632781109776782813014506245963275432586669921875;-0.662040518236455266531947927433066070079803466796875;-0.3140604546433773958113988555851392447948455810546875]
      mask Display: e = 0.06;c1 = [120 150 230]/255;c2 = ([120 150 230]+0)/383;c3 = ([120 150 230]+128)/383;patch([0 1 1 0],[0 0 1 1],c1);patch([0 1 1 1-e 1-e 0+e],[0 0 1 1-e 0+e 0+e],c2);patch([0 0 1 1-e 0+e 0+e],[0 1 1 1-e 1-e 0+e],c3);plot([0 1 1 0 0],[0 0 1 1 0]);disp('Weights');
  "IW{1,1}(57,:)'" : Constant  Value=[-0.788236189356705807540492969565093517303466796875;-0.1696796842000009297724005818963632918894290924072265625;0.6417670522616527595261004535132087767124176025390625;0.89503942918971535203098710553604178130626678466796875;-0.77966013415553969689852920055272988975048065185546875;1.27105310230965340423381348955444991588592529296875;-0.46215764320585839275423722938285209238529205322265625;-0.0405008717360720582600919215110479854047298431396484375]
      mask Display: e = 0.06;c1 = [120 150 230]/255;c2 = ([120 150 230]+0)/383;c3 = ([120 150 230]+128)/383;patch([0 1 1 0],[0 0 1 1],c1);patch([0 1 1 1-e 1-e 0+e],[0 0 1 1-e 0+e 0+e],c2);patch([0 0 1 1-e 0+e 0+e],[0 1 1 1-e 1-e 0+e],c3);plot([0 1 1 0 0],[0 0 1 1 0]);disp('Weights');
  "IW{1,1}(58,:)'" : Constant  Value=[-0.282776919567824081003237779441406019032001495361328125;0.55475339132254342100480926092131994664669036865234375;0.131770063646997226403101421965402550995349884033203125;-0.69602911123392086079064711157116107642650604248046875;0.7047800121582998844615985944983549416065216064453125;1.1977953547179989168824931766721419990062713623046875;-0.006867101369382916202510624970045682857744395732879638671875;0.52127151069329091814807952687260694801807403564453125]
      mask Display: e = 0.06;c1 = [120 150 230]/255;c2 = ([120 150 230]+0)/383;c3 = ([120 150 230]+128)/383;patch([0 1 1 0],[0 0 1 1],c1);patch([0 1 1 1-e 1-e 0+e],[0 0 1 1-e 0+e 0+e],c2);patch([0 0 1 1-e 0+e 0+e],[0 1 1 1-e 1-e 0+e],c3);plot([0 1 1 0 0],[0 0 1 1 0]);disp('Weights');
  "IW{1,1}(59,:)'" : Constant  Value=[-1.32280200133149516972252968116663396358489990234375;-1.241498673040075662044046111986972391605377197265625;0.1112030233925446476295206821305328048765659332275390625;-0.0949003654198495583127481722840457223355770111083984375;0.5853047141479397197372236405499279499053955078125;-1.2034558547379912152308634176733903586864471435546875;0.8571376516073903051307070199982263147830963134765625;-0.356667365021951232595398550984100438654422760009765625]
      mask Display: e = 0.06;c1 = [120 150 230]/255;c2 = ([120 150 230]+0)/383;c3 = ([120 150 230]+128)/383;patch([0 1 1 0],[0 0 1 1],c1);patch([0 1 1 1-e 1-e 0+e],[0 0 1 1-e 0+e 0+e],c2);patch([0 0 1 1-e 0+e 0+e],[0 1 1 1-e 1-e 0+e],c3);plot([0 1 1 0 0],[0 0 1 1 0]);disp('Weights');
  "IW{1,1}(6,:)'" : Constant  Value=[-0.647641582751347311130984962801449000835418701171875;-0.05389082719843975299855998173370608128607273101806640625;0.72723263072112731553175990484305657446384429931640625;0.642663017785146006843888244475238025188446044921875;0.60355377753536865181871462482376955449581146240234375;1.216413729119398823286246624775230884552001953125;-0.332393094321415005776287898697773925960063934326171875;0.6742071058142133921364802517928183078765869140625]
      mask Display: e = 0.06;c1 = [120 150 230]/255;c2 = ([120 150 230]+0)/383;c3 = ([120 150 230]+128)/383;patch([0 1 1 0],[0 0 1 1],c1);patch([0 1 1 1-e 1-e 0+e],[0 0 1 1-e 0+e 0+e],c2);patch([0 0 1 1-e 0+e 0+e],[0 1 1 1-e 1-e 0+e],c3);plot([0 1 1 0 0],[0 0 1 1 0]);disp('Weights');
  "IW{1,1}(60,:)'" : Constant  Value=[-0.29841697320189186637406919544446282088756561279296875;0.1751102111160622865071445630746893584728240966796875;-0.56120483503503171274218175312853418290615081787109375;-1.1526376573287977489457034607767127454280853271484375;-0.7796632550440090181353980369749478995800018310546875;1.1103602153930136609005785430781543254852294921875;1.29675686533358724972231357241980731487274169921875;0.256630224564948772325578829622827470302581787109375]
      mask Display: e = 0.06;c1 = [120 150 230]/255;c2 = ([120 150 230]+0)/383;c3 = ([120 150 230]+128)/383;patch([0 1 1 0],[0 0 1 1],c1);patch([0 1 1 1-e 1-e 0+e],[0 0 1 1-e 0+e 0+e],c2);patch([0 0 1 1-e 0+e 0+e],[0 1 1 1-e 1-e 0+e],c3);plot([0 1 1 0 0],[0 0 1 1 0]);disp('Weights');
  "IW{1,1}(61,:)'" : Constant  Value=[0.327673661172264096830275548200006596744060516357421875;-1.1852146403487981984881116659380495548248291015625;-0.8356628172465112580624690963304601609706878662109375;1.1507140513832607719990619443706236779689788818359375;0.422649337780528211450103981405845843255519866943359375;-0.90675257831490052584655359169119037687778472900390625;-0.61351513840491722628911475112545304000377655029296875;0.77068548026065053502264845519675873219966888427734375]
      mask Display: e = 0.06;c1 = [120 150 230]/255;c2 = ([120 150 230]+0)/383;c3 = ([120 150 230]+128)/383;patch([0 1 1 0],[0 0 1 1],c1);patch([0 1 1 1-e 1-e 0+e],[0 0 1 1-e 0+e 0+e],c2);patch([0 0 1 1-e 0+e 0+e],[0 1 1 1-e 1-e 0+e],c3);plot([0 1 1 0 0],[0 0 1 1 0]);disp('Weights');
  "IW{1,1}(62,:)'" : Constant  Value=[-1.01222175358292876268251347937621176242828369140625;0.30772903857483180356524599119438789784908294677734375;0.1258447111360571357696613858934142626821994781494140625;-0.2048272957368057201055222549257450737059116363525390625;1.04659222892280379113572053029201924800872802734375;-1.023650618088968844432429250446148216724395751953125;0.96149659541473264656730179922305978834629058837890625;-1.0691683282896826678864954374148510396480560302734375]
      mask Display: e = 0.06;c1 = [120 150 230]/255;c2 = ([120 150 230]+0)/383;c3 = ([120 150 230]+128)/383;patch([0 1 1 0],[0 0 1 1],c1);patch([0 1 1 1-e 1-e 0+e],[0 0 1 1-e 0+e 0+e],c2);patch([0 0 1 1-e 0+e 0+e],[0 1 1 1-e 1-e 0+e],c3);plot([0 1 1 0 0],[0 0 1 1 0]);disp('Weights');
  "IW{1,1}(63,:)'" : Constant  Value=[0.195546427152749668909592628551763482391834259033203125;0.2287492720815610114382110396036296151578426361083984375;0.86134122089192366455989713358576409518718719482421875;-1.048306188726943588562789955176413059234619140625;0.9216840303458671002090341062285006046295166015625;0.464502666454476076385304850191459991037845611572265625;-1.46095669606850275812348627368919551372528076171875;0.04961753802036659999341594584620906971395015716552734375]
      mask Display: e = 0.06;c1 = [120 150 230]/255;c2 = ([120 150 230]+0)/383;c3 = ([120 150 230]+128)/383;patch([0 1 1 0],[0 0 1 1],c1);patch([0 1 1 1-e 1-e 0+e],[0 0 1 1-e 0+e 0+e],c2);patch([0 0 1 1-e 0+e 0+e],[0 1 1 1-e 1-e 0+e],c3);plot([0 1 1 0 0],[0 0 1 1 0]);disp('Weights');
  "IW{1,1}(64,:)'" : Constant  Value=[-1.341647093590799588724848945275880396366119384765625;0.494386557133207060754642725441954098641872406005859375;-0.9742833195380529165419147830107249319553375244140625;-0.490145582947635272130781913801911287009716033935546875;0.283693624328360705089124849109794013202190399169921875;1.222641006826332699120030156336724758148193359375;0.463857209333898234948634353713714517652988433837890625;0.69672386098843730461993573044310323894023895263671875]
      mask Display: e = 0.06;c1 = [120 150 230]/255;c2 = ([120 150 230]+0)/383;c3 = ([120 150 230]+128)/383;patch([0 1 1 0],[0 0 1 1],c1);patch([0 1 1 1-e 1-e 0+e],[0 0 1 1-e 0+e 0+e],c2);patch([0 0 1 1-e 0+e 0+e],[0 1 1 1-e 1-e 0+e],c3);plot([0 1 1 0 0],[0 0 1 1 0]);disp('Weights');
  "IW{1,1}(7,:)'" : Constant  Value=[-0.6441223072216717415727771367528475821018218994140625;1.2024127442640304419541052993736229836940765380859375;1.190542341822362626402309615514241158962249755859375;-0.14559750450257469278625421793549321591854095458984375;-0.348178053061322378969322244302020408213138580322265625;-1.2120394474561699826864469287102110683917999267578125;0.0078193818859832731060777177845011465251445770263671875;0.703317217437139152735880998079665005207061767578125]
      mask Display: e = 0.06;c1 = [120 150 230]/255;c2 = ([120 150 230]+0)/383;c3 = ([120 150 230]+128)/383;patch([0 1 1 0],[0 0 1 1],c1);patch([0 1 1 1-e 1-e 0+e],[0 0 1 1-e 0+e 0+e],c2);patch([0 0 1 1-e 0+e 0+e],[0 1 1 1-e 1-e 0+e],c3);plot([0 1 1 0 0],[0 0 1 1 0]);disp('Weights');
  "IW{1,1}(8,:)'" : Constant  Value=[-1.2130180218773325417913611090625636279582977294921875;0.058317907292045896572307839278437313623726367950439453125;-0.7224555011965236861470884832669980823993682861328125;-1.1361547906194224832887584852869622409343719482421875;-1.01205039212307834617377011454664170742034912109375;0.1290720124879272956430753538370481692254543304443359375;-0.0358768950798835362103744728301535360515117645263671875;0.555346756087708559590510049019940197467803955078125]
      mask Display: e = 0.06;c1 = [120 150 230]/255;c2 = ([120 150 230]+0)/383;c3 = ([120 150 230]+128)/383;patch([0 1 1 0],[0 0 1 1],c1);patch([0 1 1 1-e 1-e 0+e],[0 0 1 1-e 0+e 0+e],c2);patch([0 0 1 1-e 0+e 0+e],[0 1 1 1-e 1-e 0+e],c3);plot([0 1 1 0 0],[0 0 1 1 0]);disp('Weights');
  "IW{1,1}(9,:)'" : Constant  Value=[-0.91891166932257017929686071511241607367992401123046875;-0.15606431575632206953940794846857897937297821044921875;0.34514558439929832189818625920452177524566650390625;0.2520813370518493190530762149137444794178009033203125;0.2868699278029815946666758463834412395954132080078125;0.44610088839530970261648690211586654186248779296875;1.3524209604642096760329650351195596158504486083984375;-0.98565174866429716704629981904872693121433258056640625]
      mask Display: e = 0.06;c1 = [120 150 230]/255;c2 = ([120 150 230]+0)/383;c3 = ([120 150 230]+128)/383;patch([0 1 1 0],[0 0 1 1],c1);patch([0 1 1 1-e 1-e 0+e],[0 0 1 1-e 0+e 0+e],c2);patch([0 0 1 1-e 0+e 0+e],[0 1 1 1-e 1-e 0+e],c3);plot([0 1 1 0 0],[0 0 1 1 0]);disp('Weights');
  Mux : Mux  Inputs=64
      mask Display: e = 0.06;c1 = [120 150 230]/255;c2 = ([120 150 230]+0)/383;c3 = ([120 150 230]+128)/383;patch([0 1 1 0],[0 0 1 1],c1);patch([0 1 1 1-e 1-e 0+e],[0 0 1 1-e 0+e 0+e],c2);patch([0 0 1 1-e 0+e 0+e],[0 1 1 1-e 1-e 0+e],c3);plot([0 1 1 0 0],[0 0 1 1 0]);disp('Mux');
  dotprod{1..64} (64 alike) : neural/Weight Functions/dotprod
  "iz{1,1}" : Outport
      mask Display: e = 0.06;c1 = [120 230 180]/255;c2 = ([120 230 180]+0)/(256+128);c3 = ([120 230 180]+128)/(256+128);patch([0 1 1 0],[0 0 1 1],c1);patch([0 1 1 1-e 1-e 0+e],[0 0 1 1-e 0+e 0+e],c2);patch([0 0 1 1-e 0+e 0+e],[0 1 1 1-e 1-e 0+e],c3);plot([0 1 1 0 0],[0 0 1 1 0]);
  wires:
  "IW{1,1}(1,:)'"/1 -> dotprod1/1
  "pd{1,1}"/1 -> dotprod1/2, dotprod2/2, dotprod3/2, dotprod4/2, dotprod5/2, dotprod6/2, dotprod7/2, dotprod8/2, dotprod9/2, dotprod10/2, dotprod11/2, dotprod12/2, dotprod13/2, dotprod14/2, dotprod15/2, dotprod16/2, dotprod17/2, dotprod18/2, dotprod19/2, dotprod20/2, dotprod21/2, dotprod22/2, dotprod23/2, dotprod24/2, dotprod25/2, dotprod26/2, dotprod27/2, dotprod28/2, dotprod29/2, dotprod30/2, dotprod31/2, dotprod32/2, dotprod33/2, dotprod34/2, dotprod35/2, dotprod36/2, dotprod37/2, dotprod38/2, dotprod39/2, dotprod40/2, dotprod41/2, dotprod42/2, dotprod43/2, dotprod44/2, dotprod45/2, dotprod46/2, dotprod47/2, dotprod48/2, dotprod49/2, dotprod50/2, dotprod51/2, dotprod52/2, dotprod53/2, dotprod54/2, dotprod55/2, dotprod56/2, dotprod57/2, dotprod58/2, dotprod59/2, dotprod60/2, dotprod61/2, dotprod62/2, dotprod63/2, dotprod64/2
  dotprod1/1 -> Mux/1
  "IW{1,1}(2,:)'"/1 -> dotprod2/1
  dotprod2/1 -> Mux/2
  "IW{1,1}(3,:)'"/1 -> dotprod3/1
  dotprod3/1 -> Mux/3
  "IW{1,1}(4,:)'"/1 -> dotprod4/1
  dotprod4/1 -> Mux/4
  "IW{1,1}(5,:)'"/1 -> dotprod5/1
  dotprod5/1 -> Mux/5
  "IW{1,1}(6,:)'"/1 -> dotprod6/1
  dotprod6/1 -> Mux/6
  "IW{1,1}(7,:)'"/1 -> dotprod7/1
  dotprod7/1 -> Mux/7
  "IW{1,1}(8,:)'"/1 -> dotprod8/1
  dotprod8/1 -> Mux/8
  "IW{1,1}(9,:)'"/1 -> dotprod9/1
  dotprod9/1 -> Mux/9
  "IW{1,1}(10,:)'"/1 -> dotprod10/1
  dotprod10/1 -> Mux/10
  "IW{1,1}(11,:)'"/1 -> dotprod11/1
  dotprod11/1 -> Mux/11
  "IW{1,1}(12,:)'"/1 -> dotprod12/1
  dotprod12/1 -> Mux/12
  "IW{1,1}(13,:)'"/1 -> dotprod13/1
  dotprod13/1 -> Mux/13
  "IW{1,1}(14,:)'"/1 -> dotprod14/1
  dotprod14/1 -> Mux/14
  "IW{1,1}(15,:)'"/1 -> dotprod15/1
  dotprod15/1 -> Mux/15
  "IW{1,1}(16,:)'"/1 -> dotprod16/1
  dotprod16/1 -> Mux/16
  "IW{1,1}(17,:)'"/1 -> dotprod17/1
  dotprod17/1 -> Mux/17
  "IW{1,1}(18,:)'"/1 -> dotprod18/1
  dotprod18/1 -> Mux/18
  "IW{1,1}(19,:)'"/1 -> dotprod19/1
  dotprod19/1 -> Mux/19
  "IW{1,1}(20,:)'"/1 -> dotprod20/1
  dotprod20/1 -> Mux/20
  "IW{1,1}(21,:)'"/1 -> dotprod21/1
  dotprod21/1 -> Mux/21
  "IW{1,1}(22,:)'"/1 -> dotprod22/1
  dotprod22/1 -> Mux/22
  "IW{1,1}(23,:)'"/1 -> dotprod23/1
  dotprod23/1 -> Mux/23
  "IW{1,1}(24,:)'"/1 -> dotprod24/1
  dotprod24/1 -> Mux/24
  "IW{1,1}(25,:)'"/1 -> dotprod25/1
  dotprod25/1 -> Mux/25
  "IW{1,1}(26,:)'"/1 -> dotprod26/1
  dotprod26/1 -> Mux/26
  "IW{1,1}(27,:)'"/1 -> dotprod27/1
  dotprod27/1 -> Mux/27
  "IW{1,1}(28,:)'"/1 -> dotprod28/1
  dotprod28/1 -> Mux/28
  "IW{1,1}(29,:)'"/1 -> dotprod29/1
  dotprod29/1 -> Mux/29
  "IW{1,1}(30,:)'"/1 -> dotprod30/1
  dotprod30/1 -> Mux/30
  "IW{1,1}(31,:)'"/1 -> dotprod31/1
  dotprod31/1 -> Mux/31
  "IW{1,1}(32,:)'"/1 -> dotprod32/1
  dotprod32/1 -> Mux/32
  "IW{1,1}(33,:)'"/1 -> dotprod33/1
  dotprod33/1 -> Mux/33
  "IW{1,1}(34,:)'"/1 -> dotprod34/1
  dotprod34/1 -> Mux/34
  "IW{1,1}(35,:)'"/1 -> dotprod35/1
  dotprod35/1 -> Mux/35
  "IW{1,1}(36,:)'"/1 -> dotprod36/1
  dotprod36/1 -> Mux/36
  "IW{1,1}(37,:)'"/1 -> dotprod37/1
  dotprod37/1 -> Mux/37
  "IW{1,1}(38,:)'"/1 -> dotprod38/1
  dotprod38/1 -> Mux/38
  "IW{1,1}(39,:)'"/1 -> dotprod39/1
  dotprod39/1 -> Mux/39
  "IW{1,1}(40,:)'"/1 -> dotprod40/1
  dotprod40/1 -> Mux/40
  "IW{1,1}(41,:)'"/1 -> dotprod41/1
  dotprod41/1 -> Mux/41
  "IW{1,1}(42,:)'"/1 -> dotprod42/1
  dotprod42/1 -> Mux/42
  "IW{1,1}(43,:)'"/1 -> dotprod43/1
  dotprod43/1 -> Mux/43
  "IW{1,1}(44,:)'"/1 -> dotprod44/1
  dotprod44/1 -> Mux/44
  "IW{1,1}(45,:)'"/1 -> dotprod45/1
  dotprod45/1 -> Mux/45
  "IW{1,1}(46,:)'"/1 -> dotprod46/1
  dotprod46/1 -> Mux/46
  "IW{1,1}(47,:)'"/1 -> dotprod47/1
  dotprod47/1 -> Mux/47
  "IW{1,1}(48,:)'"/1 -> dotprod48/1
  dotprod48/1 -> Mux/48
  "IW{1,1}(49,:)'"/1 -> dotprod49/1
  dotprod49/1 -> Mux/49
  "IW{1,1}(50,:)'"/1 -> dotprod50/1
  dotprod50/1 -> Mux/50
  "IW{1,1}(51,:)'"/1 -> dotprod51/1
  dotprod51/1 -> Mux/51
  "IW{1,1}(52,:)'"/1 -> dotprod52/1
  dotprod52/1 -> Mux/52
  "IW{1,1}(53,:)'"/1 -> dotprod53/1
  dotprod53/1 -> Mux/53
  "IW{1,1}(54,:)'"/1 -> dotprod54/1
  dotprod54/1 -> Mux/54
  "IW{1,1}(55,:)'"/1 -> dotprod55/1
  dotprod55/1 -> Mux/55
  "IW{1,1}(56,:)'"/1 -> dotprod56/1
  dotprod56/1 -> Mux/56
  "IW{1,1}(57,:)'"/1 -> dotprod57/1
  dotprod57/1 -> Mux/57
  "IW{1,1}(58,:)'"/1 -> dotprod58/1
  dotprod58/1 -> Mux/58
  "IW{1,1}(59,:)'"/1 -> dotprod59/1
  dotprod59/1 -> Mux/59
  "IW{1,1}(60,:)'"/1 -> dotprod60/1
  dotprod60/1 -> Mux/60
  "IW{1,1}(61,:)'"/1 -> dotprod61/1
  dotprod61/1 -> Mux/61
  "IW{1,1}(62,:)'"/1 -> dotprod62/1
  dotprod62/1 -> Mux/62
  "IW{1,1}(63,:)'"/1 -> dotprod63/1
  dotprod63/1 -> Mux/63
  "IW{1,1}(64,:)'"/1 -> dotprod64/1
  dotprod64/1 -> Mux/64
  Mux/1 -> "iz{1,1}"/1
